simulink model "zadacha_19_model"  (Simulink 7.1)
settings: Solver=ode45  StartTime=0.0  StopTime=200  RelTol=1e-3
values from neighbouring files (symbols this model uses):
  D = fp(3)    [pidfunc.m]
  I = fp(2)    [pidfunc.m]
  P = fp(1)    [pidfunc.m]
settings Model: Creator=Slavi  LastModifiedBy=Slavi

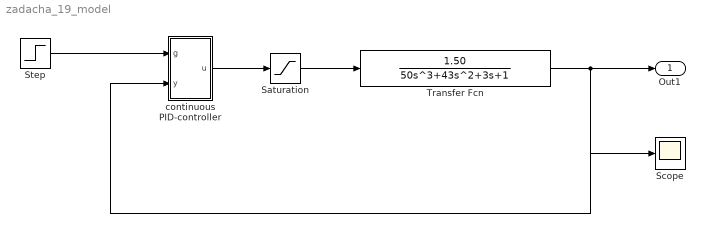
== system zadacha_19_model ==
  Saturation : Saturate  UpperLimit=2  LowerLimit=-2  OutDataType=sfix(16)  OutScaling=2^0
  Scope : Scope
  Step : Step  Time=0
  Transfer Fcn : TransferFcn  Numerator=[1.50]  Denominator=[50 43 3 1]
  continuous PID-controller : Subsystem  mask(PID_REG_continuous){P=P, I=I, D=D}
      mask prompts: P "P="; I "I="; D "D="
      mask help: PID continuous regulator
      mask init:
      | q0=P;
      | q1=P/I;
      | q2=P*D;
      mask Help: enter P, I, D
  Out1 : Outport  OutDataType=sfix(16)  OutScaling=2^0
  wires:
  Transfer Fcn/1 -> Out1/1, Scope/1, continuous PID-controller/2(y)
  Step/1 -> continuous PID-controller/1(g)
  continuous PID-controller/1(u) -> Saturation/1
  Saturation/1 -> Transfer Fcn/1

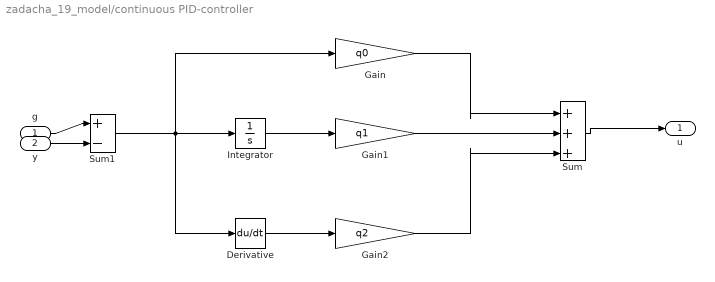
== system zadacha_19_model/continuous PID-controller ==
  g : Inport
  y : Inport  Port=2
  Derivative : Derivative
  Gain : Gain  Gain=q0  ParameterDataType=sfix(16)  ParameterScaling=2^0  OutDataType=sfix(16)  OutScaling=2^0
  Gain1 : Gain  Gain=q1  ParameterDataType=sfix(16)  ParameterScaling=2^0  OutDataType=sfix(16)  OutScaling=2^0
  Gain2 : Gain  Gain=q2  ParameterDataType=sfix(16)  ParameterScaling=2^0  OutDataType=sfix(16)  OutScaling=2^0
  Integrator : Integrator
  Sum : Sum  Inputs=|+++  OutDataType=sfix(16)  OutScaling=2^0
  Sum1 : Sum  Inputs=|+-  OutDataType=sfix(16)  OutScaling=2^0
  u : Outport  OutDataType=sfix(16)  OutScaling=2^0
  wires:
  Integrator/1 -> Gain1/1
  Derivative/1 -> Gain2/1
  Gain1/1 -> Sum/2
  Gain2/1 -> Sum/3
  Gain/1 -> Sum/1
  Sum1/1 -> Gain/1, Derivative/1, Integrator/1
  y/1 -> Sum1/2
  g/1 -> Sum1/1
  Sum/1 -> u/1
